simulink model "momentumBasedFlying"  (Simulink 9.0)
settings: Solver=FixedStepAuto  StartTime=0.0  StopTime="Config.simulationTime "  FixedStep=Config.Ts  RelTol=1e-3  EnableMultiTasking=on
InitFcn:
  | cd(fileparts(which(bdroot)));
  | initMomentumBasedFlying;
StopFcn:
  | visualizer_demo_idyntree(time.Data,state.Data,Config,desired_x_dx_ddx_dddx_CoM,jetsIntensitiesByWeight);
undefined symbols (not defined in the file or in its folder): Config, config
libraries: WBToolboxLibrary x67, simulink x2
(part 1 of 2)
settings Model: SuppressorTable=22 serialization::archive 11 0 6 0 0 0 11 0  Creator=DanielePucci  LastModifiedBy=gnava
settings DataIOCC: LimitDataPoints=on  SaveFormat=Dataset
settings DebuggingCC: UnderspecifiedInitializationDetection=Simplified  MergeDetectMultiDrivingBlocksExec=error  AllowSymbolicDim=off
settings HardwareCC: ProdBitPerPointer=64  ProdBitPerSizeT=64  ProdBitPerPtrDiffT=64  ProdLargestAtomicFloat=Float  ProdIntDivRoundTo=Zero  ProdEndianess=LittleEndian  ProdWordSize=64  ProdHWDeviceType=Intel->x86-64 (Windows64)

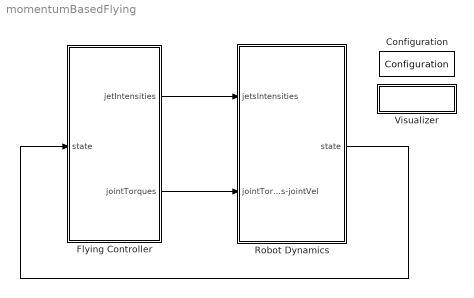
== system momentumBasedFlying ==
  Configuration : WBToolboxLibrary/Utilities/Configuration  ConfigSource=Workspace  ConfigObject='WBTConfigRobot'
      settings: SourceProductName=Whole Body Toolbox
  Flying Controller : Subsystem
  Robot Dynamics : Subsystem
  Visualizer : Subsystem
      mask Display: disp('Visualizer');
  wires:
  Flying Controller/1(jetIntensities) -> Robot Dynamics/1(jetsIntensities)
  Flying Controller/2(jointTorques) -> Robot Dynamics/2(jointTorques-jointVel)
  Robot Dynamics/1(state) -> Flying Controller/1(state)

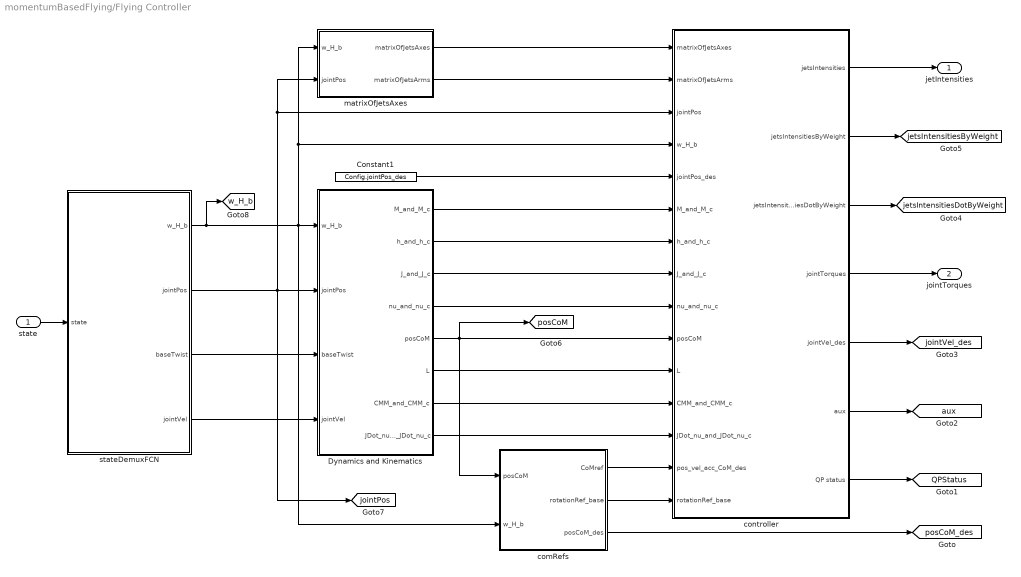
== system momentumBasedFlying/Flying Controller ==
  state : Inport
  Constant1 : Constant  Value=Config.jointPos_des
  Dynamics and Kinematics : Subsystem
  comRefs : Subsystem
  controller : Subsystem
  matrixOfJetsAxes : Subsystem
  stateDemuxFCN : MATLAB Function  TreatAsAtomicUnit=on
  jetIntensities : Outport
  jointTorques : Outport  Port=2
  tag scope: QPStatus=global, aux=global, jetsIntensitiesByWeight=global, jetsIntensitiesDotByWeight=global, jointPos=global, jointVel_des=global, posCoM=global, posCoM_des=global, w_H_b=global
  wires:
  state/1 -> stateDemuxFCN/1(state)
  controller/4(jointTorques) -> jointTorques/1
  controller/1(jetsIntensities) -> jetIntensities/1
  stateDemuxFCN/4(jointVel) -> Dynamics and Kinematics/4(jointVel)
  stateDemuxFCN/3(baseTwist) -> Dynamics and Kinematics/3(baseTwist)
  stateDemuxFCN/2(jointPos) -> [jointPos], matrixOfJetsAxes/2(jointPos), controller/3(jointPos), Dynamics and Kinematics/2(jointPos)
  stateDemuxFCN/1(w_H_b) -> comRefs/2(w_H_b), matrixOfJetsAxes/1(w_H_b), controller/4(w_H_b), Dynamics and Kinematics/1(w_H_b), [w_H_b]
  Dynamics and Kinematics/1(M_and_M_c) -> controller/6(M_and_M_c)
  Dynamics and Kinematics/2(h_and_h_c) -> controller/7(h_and_h_c)
  Dynamics and Kinematics/3(J_and_J_c) -> controller/8(J_and_J_c)
  Dynamics and Kinematics/4(nu_and_nu_c) -> controller/9(nu_and_nu_c)
  Dynamics and Kinematics/5(posCoM) -> [posCoM], comRefs/1(posCoM), controller/10(posCoM)
  Dynamics and Kinematics/6(L) -> controller/11(L)
  Dynamics and Kinematics/7(CMM_and_CMM_c) -> controller/12(CMM_and_CMM_c)
  Dynamics and Kinematics/8(JDot_nu_and_JDot_nu_c) -> controller/13(JDot_nu_and_JDot_nu_c)
  matrixOfJetsAxes/1(matrixOfJetsAxes) -> controller/1(matrixOfJetsAxes)
  matrixOfJetsAxes/2(matrixOfJetsArms) -> controller/2(matrixOfJetsArms)
  Constant1/1 -> controller/5(jointPos_des)
  comRefs/1(CoMref) -> controller/14(pos_vel_acc_CoM_des)
  comRefs/2(rotationRef_base) -> controller/15(rotationRef_base)
  comRefs/3(posCoM_des) -> [posCoM_des]
  controller/2(jetsIntensitiesByWeight) -> [jetsIntensitiesByWeight]
  controller/3(jetsIntensitiesDotByWeight) -> [jetsIntensitiesDotByWeight]
  controller/5(jointVel_des) -> [jointVel_des]
  controller/6(aux) -> [aux]
  controller/7(QP status) -> [QPStatus]

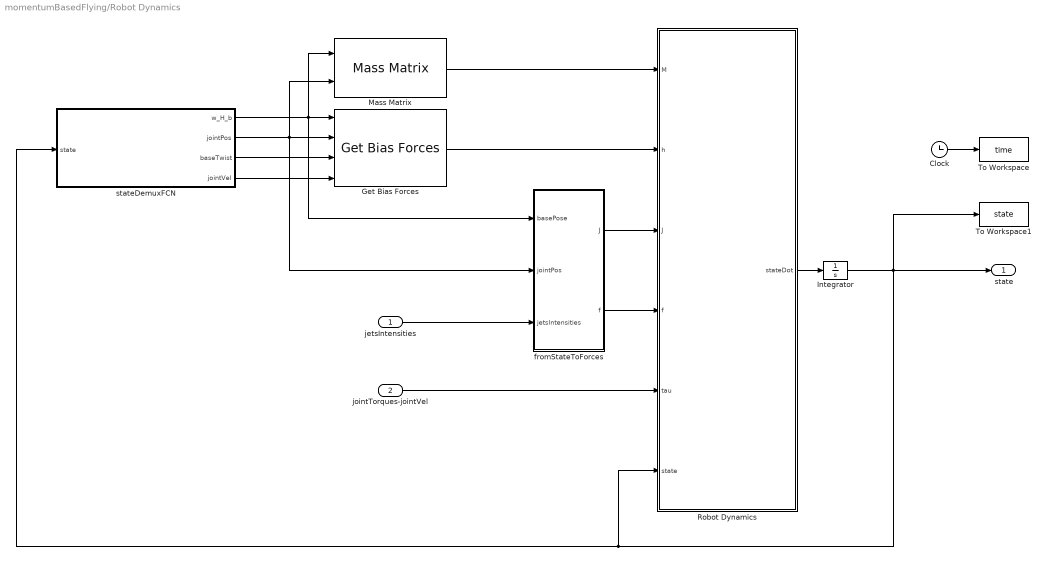
== system momentumBasedFlying/Robot Dynamics ==
  jetsIntensities : Inport
  jointTorques-jointVel : Inport  Port=2
  Clock : Clock
  Get Bias Forces : WBToolboxLibrary/wholeBodyModel/Dynamics/Get Bias Forces
      settings: SourceProductName=Whole Body Toolbox
  Integrator : Integrator  InitialCondition=Config.initState
  Mass Matrix : WBToolboxLibrary/wholeBodyModel/Dynamics/Mass Matrix
      settings: SourceProductName=Whole Body Toolbox
  Robot Dynamics : MATLAB Function  TreatAsAtomicUnit=on
  To Workspace : ToWorkspace  VariableName=time  SaveFormat=Timeseries  SampleTime=-1
  To Workspace1 : ToWorkspace  VariableName=state  SaveFormat=Timeseries  SampleTime=-1
  fromStateToForces : Subsystem
  stateDemuxFCN : MATLAB Function  TreatAsAtomicUnit=on
  state : Outport
  wires:
  Robot Dynamics/1(stateDot) -> Integrator/1
  jointTorques-jointVel/1 -> Robot Dynamics/5(tau)
  stateDemuxFCN/4(jointVel) -> Get Bias Forces/4
  stateDemuxFCN/2(jointPos) -> fromStateToForces/2(jointPos), Get Bias Forces/2, Mass Matrix/2
  stateDemuxFCN/1(w_H_b) -> fromStateToForces/1(basePose), Get Bias Forces/1, Mass Matrix/1
  stateDemuxFCN/3(baseTwist) -> Get Bias Forces/3
  Mass Matrix/1 -> Robot Dynamics/1(M)
  Get Bias Forces/1 -> Robot Dynamics/2(h)
  jetsIntensities/1 -> fromStateToForces/3(jetsIntensities)
  fromStateToForces/1(J) -> Robot Dynamics/3(J)
  fromStateToForces/2(f) -> Robot Dynamics/4(f)
  Integrator/1 -> To Workspace1/1, state/1, Robot Dynamics/6(state), stateDemuxFCN/1(state)
  Clock/1 -> To Workspace/1

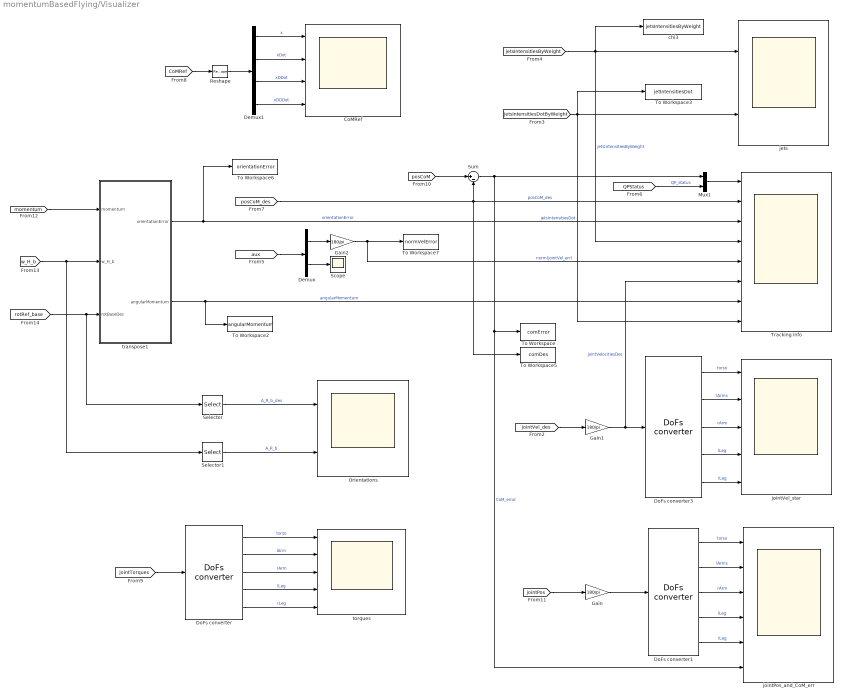
== system momentumBasedFlying/Visualizer ==
  CoMRef : Scope  NumInputPorts=4
  Demux : Demux  Outputs=2
  Demux1 : Demux  Outputs=[3;3;3;3]
  DoFs converter : WBToolboxLibrary/Utilities/DoFs converter  yarp2WBIOption=From YARP to WBI
      settings: SourceProductName=Whole Body Toolbox
  DoFs converter1 : WBToolboxLibrary/Utilities/DoFs converter  yarp2WBIOption=From YARP to WBI
      settings: SourceProductName=Whole Body Toolbox
  DoFs converter3 : WBToolboxLibrary/Utilities/DoFs converter  yarp2WBIOption=From YARP to WBI
      settings: SourceProductName=Whole Body Toolbox
  Gain : Gain  Gain=180/pi
  Gain1 : Gain  Gain=180/pi
  Gain2 : Gain  Gain=180/pi
  Mux1 : Mux  Inputs=2
  Orientations : Scope  NumInputPorts=2
  Reshape : Reshape
  Scope : Scope
  Selector : Selector  NumberOfDimensions=2  InputPortWidth=3  IndexOptions=Index vector (dialog),Index vector (dialog)  Indices=[1 2 3],[1 2 3]  OutputSizes=1,1
  Selector1 : Selector  NumberOfDimensions=2  InputPortWidth=3  IndexOptions=Index vector (dialog),Index vector (dialog)  Indices=[1 2 3],[1 2 3]  OutputSizes=1,1
  Sum : Sum  Inputs=|+-
  To Workspace : ToWorkspace  VariableName=comError  SaveFormat=Timeseries  SampleTime=-1
  To Workspace2 : ToWorkspace  VariableName=angularMomentum  SaveFormat=Timeseries  SampleTime=-1
  To Workspace3 : ToWorkspace  VariableName=jetIntensitiesDot  SaveFormat=Timeseries  SampleTime=-1
  To Workspace5 : ToWorkspace  VariableName=comDes  SaveFormat=Timeseries  SampleTime=-1
  To Workspace6 : ToWorkspace  VariableName=orientationError  SaveFormat=Timeseries  SampleTime=-1
  To Workspace7 : ToWorkspace  VariableName=normVelError  SaveFormat=Timeseries  SampleTime=-1
  Tracking info : Scope  NumInputPorts=8
  chi3 : ToWorkspace  VariableName=jetsIntensitiesByWeight  SaveFormat=Timeseries  SampleTime=-1
  jets : Scope  NumInputPorts=2
  jointPos_and_CoM_err : Scope  NumInputPorts=6
  jointVel_star : Scope  NumInputPorts=5
  torques : Scope  NumInputPorts=5
  transpose1 : MATLAB Function  TreatAsAtomicUnit=on
  wires:
  Demux/1 -> Gain2/1
  DoFs converter1/5 -> jointPos_and_CoM_err/5  "rLeg"
  DoFs converter/2 -> torques/2  "lArm"
  Mux1/1 -> Tracking info/1
  DoFs converter/1 -> torques/1  "torso"
  DoFs converter/5 -> torques/5  "rLeg"
  DoFs converter/3 -> torques/3  "rArm"
  DoFs converter1/3 -> jointPos_and_CoM_err/3  "rArm"
  Gain1/1 -> Tracking info/6, DoFs converter3/1  "jointVelocitiesDes"
  DoFs converter1/1 -> jointPos_and_CoM_err/1  "torso"
  [jointVel_des] -> Gain1/1
  DoFs converter3/3 -> jointVel_star/3  "rArm"
  Gain2/1 -> Tracking info/5, To Workspace7/1  "norm(jointVel_err)"
  Demux/2 -> Scope/1
  transpose1/1(orientationError) -> To Workspace6/1, Tracking info/3  "orientationError"
  Gain/1 -> DoFs converter1/1
  [aux] -> Demux/1
  DoFs converter3/1 -> jointVel_star/1  "torso"
  [jetsIntensitiesDotByWeight] -> Tracking info/8, jets/2, To Workspace3/1  "jetsIntensitiesDot"
  [jetsIntensitiesByWeight] -> Tracking info/4, chi3/1, jets/1  "jetsIntensitiesByWeight"
  DoFs converter3/2 -> jointVel_star/2  "lArms"
  DoFs converter/4 -> torques/4  "lLeg"
  [jointTorques] -> DoFs converter/1
  transpose1/2(angularMomentum) -> Tracking info/7, To Workspace2/1  "angularMomentum"
  DoFs converter3/4 -> jointVel_star/4  "lLeg"
  DoFs converter1/2 -> jointPos_and_CoM_err/2  "lArms"
  Sum/1 -> Mux1/1, jointPos_and_CoM_err/6, To Workspace/1  "CoM_error"
  DoFs converter1/4 -> jointPos_and_CoM_err/4  "lLeg"
  DoFs converter3/5 -> jointVel_star/5  "rLeg"
  [QPStatus] -> Mux1/2  "QP_status"
  Selector/1 -> Orientations/1  "A_R_b_des"
  [rotRef_base] -> Selector/1, transpose1/3(rotBaseDes)
  [w_H_b] -> Selector1/1, transpose1/2(w_H_b)
  Selector1/1 -> Orientations/2  "A_R_b"
  Demux1/4 -> CoMRef/4  "xDDDot"
  Demux1/2 -> CoMRef/2  "xDot"
  Demux1/3 -> CoMRef/3  "xDDot"
  Demux1/1 -> CoMRef/1  "x"
  [posCoM_des] -> Sum/2, To Workspace5/1, Tracking info/2  "posCoM_des"
  [CoMRef] -> Reshape/1
  Reshape/1 -> Demux1/1
  [posCoM] -> Sum/1
  [jointPos] -> Gain/1
  [momentum] -> transpose1/1(momentum)

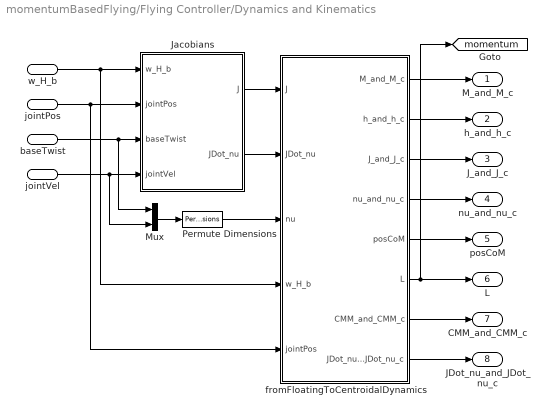
== system momentumBasedFlying/Flying Controller/Dynamics and Kinematics ==
  w_H_b : Inport
  jointPos : Inport  Port=2
  baseTwist : Inport  Port=3
  jointVel : Inport  Port=4
  Jacobians : Subsystem
  Mux : Mux  Inputs=2
  Permute Dimensions : PermuteDimensions
  fromFloatingToCentroidalDynamics : Subsystem
  M_and_M_c : Outport
  h_and_h_c : Outport  Port=2
  J_and_J_c : Outport  Port=3
  nu_and_nu_c : Outport  Port=4
  posCoM : Outport  Port=5
  L : Outport  Port=6
  CMM_and_CMM_c : Outport  Port=7
  JDot_nu_and_JDot_nu_c : Outport  Port=8
  tag scope: momentum=global
  wires:
  w_H_b/1 -> fromFloatingToCentroidalDynamics/4(w_H_b), Jacobians/1(w_H_b)
  jointPos/1 -> fromFloatingToCentroidalDynamics/5(jointPos), Jacobians/2(jointPos)
  jointVel/1 -> Mux/2, Jacobians/4(jointVel)
  baseTwist/1 -> Mux/1, Jacobians/3(baseTwist)
  Jacobians/1(J) -> fromFloatingToCentroidalDynamics/1(J)
  Mux/1 -> Permute Dimensions/1
  Jacobians/2(JDot_nu) -> fromFloatingToCentroidalDynamics/2(JDot_nu)
  Permute Dimensions/1 -> fromFloatingToCentroidalDynamics/3(nu)
  fromFloatingToCentroidalDynamics/2("h_and_h_c ") -> h_and_h_c/1
  fromFloatingToCentroidalDynamics/1(M_and_M_c) -> M_and_M_c/1
  fromFloatingToCentroidalDynamics/3(J_and_J_c) -> J_and_J_c/1
  fromFloatingToCentroidalDynamics/4(nu_and_nu_c) -> nu_and_nu_c/1
  fromFloatingToCentroidalDynamics/5(posCoM) -> posCoM/1
  fromFloatingToCentroidalDynamics/6(L) -> L/1, [momentum]
  fromFloatingToCentroidalDynamics/7(CMM_and_CMM_c) -> CMM_and_CMM_c/1
  fromFloatingToCentroidalDynamics/8(JDot_nu_and_JDot_nu_c) -> JDot_nu_and_JDot_nu_c/1

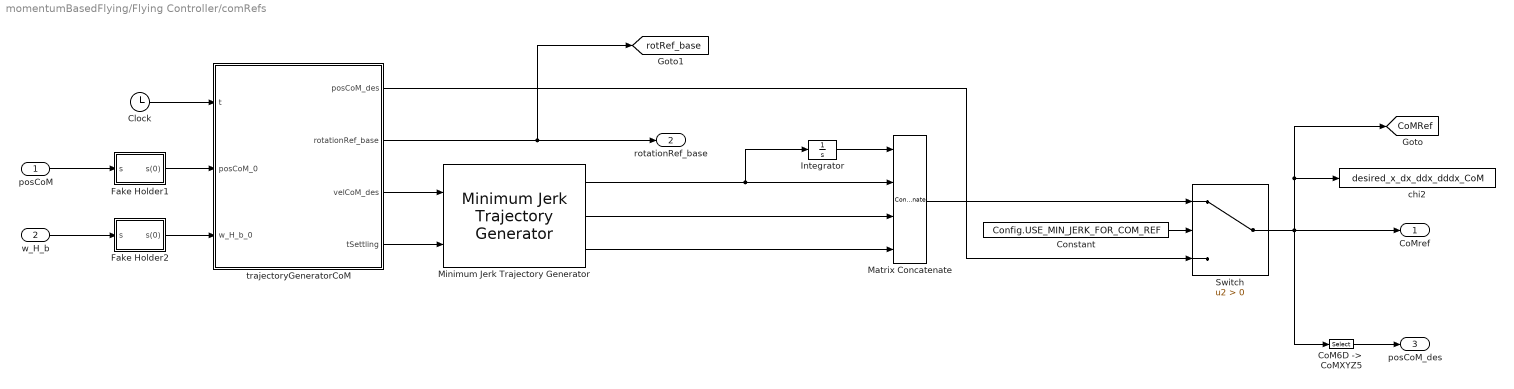
== system momentumBasedFlying/Flying Controller/comRefs ==
  posCoM : Inport
  w_H_b : Inport  Port=2
  Clock : Clock
  "CoM6D ->  CoMXYZ5" : Selector  NumberOfDimensions=2  InputPortWidth=7  IndexOptions=Index vector (dialog),Index vector (dialog)  Indices=[1 2 3],[1]  OutputSizes=1,1
  Constant : Constant  Value=Config.USE_MIN_JERK_FOR_COM_REF
  Fake Holder1 : Subsystem
  Fake Holder2 : Subsystem
  Integrator : Integrator  InitialCondition=Config.posCoM_des_0
  Matrix Concatenate : Concatenate  NumInputs=4  Mode=Multidimensional array  ConcatenateDimension=2
  Minimum Jerk Trajectory Generator : WBToolboxLibrary/Utilities/Minimum Jerk Trajectory Generator  externalSettlingTime=on  settlingTime=3  sampleTime=Config.Ts  resetOnSettlingTime=off  firstDerivatives=on  secondDerivatives=on  explicitInitialValue=off
      settings: SourceProductName=Whole Body Toolbox
  Switch : Switch  Criteria=u2 > Threshold
  chi2 : ToWorkspace  VariableName=desired_x_dx_ddx_dddx_CoM  SaveFormat=Timeseries  SampleTime=-1
  trajectoryGeneratorCoM : MATLAB Function  TreatAsAtomicUnit=on
  CoMref : Outport
  rotationRef_base : Outport  Port=2
  posCoM_des : Outport  Port=3
  tag scope: CoMRef=global, rotRef_base=global
  wires:
  Clock/1 -> trajectoryGeneratorCoM/1(t)
  trajectoryGeneratorCoM/1(posCoM_des) -> Switch/3
  posCoM/1 -> Fake Holder1/1(s)
  Fake Holder1/1(s(0)) -> trajectoryGeneratorCoM/2(posCoM_0)
  w_H_b/1 -> Fake Holder2/1(s)
  trajectoryGeneratorCoM/2(rotationRef_base) -> rotationRef_base/1, [rotRef_base]
  Fake Holder2/1(s(0)) -> trajectoryGeneratorCoM/3(w_H_b_0)
  trajectoryGeneratorCoM/3(velCoM_des) -> Minimum Jerk Trajectory Generator/1
  trajectoryGeneratorCoM/4(tSettling) -> Minimum Jerk Trajectory Generator/2
  Integrator/1 -> Matrix Concatenate/1
  Minimum Jerk Trajectory Generator/1 -> Integrator/1, Matrix Concatenate/2
  Minimum Jerk Trajectory Generator/2 -> Matrix Concatenate/3
  Minimum Jerk Trajectory Generator/3 -> Matrix Concatenate/4
  Matrix Concatenate/1 -> Switch/1
  Switch/1 -> [CoMRef], chi2/1, CoMref/1, "CoM6D ->  CoMXYZ5"/1
  Constant/1 -> Switch/2
  "CoM6D ->  CoMXYZ5"/1 -> posCoM_des/1

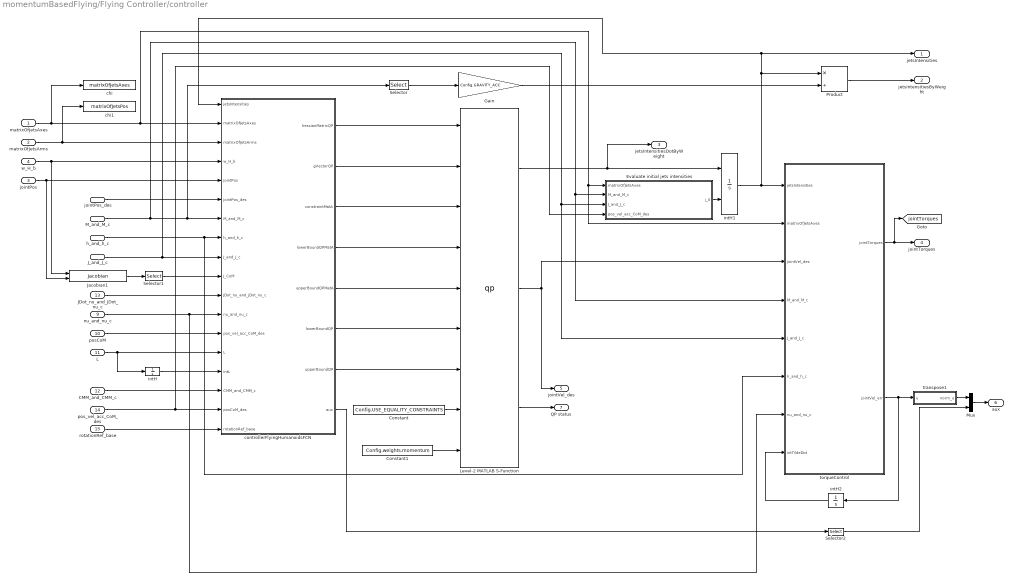
== system momentumBasedFlying/Flying Controller/controller ==
  matrixOfJetsAxes : Inport
  matrixOfJetsArms : Inport  Port=2
  jointPos : Inport  Port=3
  w_H_b : Inport  Port=4
  jointPos_des : Inport  Port=5
  M_and_M_c : Inport  Port=6
  h_and_h_c : Inport  Port=7
  J_and_J_c : Inport  Port=8
  nu_and_nu_c : Inport  Port=9
  posCoM : Inport  Port=10
  L : Inport  Port=11
  CMM_and_CMM_c : Inport  Port=12
  JDot_nu_and_JDot_nu_c : Inport  Port=13
  pos_vel_acc_CoM_des : Inport  Port=14
  rotationRef_base : Inport  Port=15
  Constant : Constant  Value=Config.USE_EQUALITY_CONSTRAINTS
  Constant1 : Constant  Value=Config.weights.momentum
  Evaluate initial jets intensities : MATLAB Function  TreatAsAtomicUnit=on
  Gain : Gain  Gain=Config.GRAVITY_ACC
  Jacobian1 : WBToolboxLibrary/wholeBodyModel/Jacobians/Jacobian  frameName=Frames.COM_FRAME
      settings: SourceProductName=Whole Body Toolbox
  Level-2 MATLAB S-Function : M-S-Function  FunctionName=qp  Parameters=Config.N_DOF  mask{ndof=Config.N_DOF}
      mask prompts: ndof "Robt degrees of freedom"
      mask Display: disp('QP')
  Mux : Mux  Inputs=2
  Product : Product  Inputs=*/
  Selector : Selector  NumberOfDimensions=2  InputPortWidth=3  IndexOptions=Index vector (dialog),Index vector (dialog)  Indices=1,1  OutputSizes=1,1
  Selector1 : Selector  NumberOfDimensions=2  InputPortWidth=3  IndexOptions=Index vector (dialog),Index vector (dialog)  Indices=[1 2 3],[1:Config.N_DOF+6]  OutputSizes=1,1
  Selector2 : Selector  InputPortWidth=2  IndexOptions=Index vector (dialog)  Indices=[2]  OutputSizes=1
  chi : ToWorkspace  VariableName=matrixOfJetsAxes  SaveFormat=Timeseries  SampleTime=-1
  chi1 : ToWorkspace  VariableName=matrixOfJetsPos  SaveFormat=Timeseries  SampleTime=-1
  controllerFlyingHumanoidsFCN : MATLAB Function  TreatAsAtomicUnit=on
  intH : Integrator  InitialCondition=zeros(6,1)
  intH1 : Integrator  InitialConditionSource=external  InitialCondition=config.jetsIntensities0
  intH2 : Integrator  InitialCondition=zeros(Config.N_DOF,1)
  torqueControl : MATLAB Function  TreatAsAtomicUnit=on
  transpose1 : MATLAB Function  TreatAsAtomicUnit=on
  jetsIntensities : Outport
  jetsIntensitiesByWeight : Outport  Port=2
  jetsIntensitiesDotByWeight : Outport  Port=3
  jointTorques : Outport  Port=4
  jointVel_des : Outport  Port=5
  aux : Outport  Port=6
  QP status : Outport  Port=7
  tag scope: jointTorques=global
  wires:
  Selector/1 -> Gain/1
  Product/1 -> jetsIntensitiesByWeight/1
  Gain/1 -> Product/2
  intH1/1 -> torqueControl/1(jetsIntensities), controllerFlyingHumanoidsFCN/1(jetsIntensities), jetsIntensities/1, Product/1
  controllerFlyingHumanoidsFCN/8(aux) -> Selector2/1
  Evaluate initial jets intensities/1(j_0) -> intH1/2
  torqueControl/1(jointTorques) -> [jointTorques], jointTorques/1
  Level-2 MATLAB S-Function/1 -> intH1/1, jetsIntensitiesDotByWeight/1
  intH2/1 -> torqueControl/8(intTildeDot)
  torqueControl/2(jointVel_err) -> intH2/1, transpose1/1(u)
  Level-2 MATLAB S-Function/2 -> jointVel_des/1, torqueControl/3(jointVel_des)
  Level-2 MATLAB S-Function/3 -> QP status/1
  Constant/1 -> Level-2 MATLAB S-Function/8
  Constant1/1 -> Level-2 MATLAB S-Function/9
  Jacobian1/1 -> Selector1/1
  Selector1/1 -> controllerFlyingHumanoidsFCN/10(J_CoM)
  Mux/1 -> aux/1
  Selector2/1 -> Mux/2
  transpose1/1(norm_u) -> Mux/1
  matrixOfJetsAxes/1 -> chi/1, controllerFlyingHumanoidsFCN/2(matrixOfJetsAxes), torqueControl/2(matrixOfJetsAxes), Evaluate initial jets intensities/1(matrixOfJetsAxes)
  matrixOfJetsArms/1 -> chi1/1, controllerFlyingHumanoidsFCN/3(matrixOfJetsArms)
  w_H_b/1 -> controllerFlyingHumanoidsFCN/4(w_H_b), Jacobian1/1
  jointPos/1 -> controllerFlyingHumanoidsFCN/5(jointPos), Jacobian1/2
  jointPos_des/1 -> controllerFlyingHumanoidsFCN/6(jointPos_des)
  M_and_M_c/1 -> controllerFlyingHumanoidsFCN/7(M_and_M_c), Selector/1, torqueControl/4(M_and_M_c), Evaluate initial jets intensities/2(M_and_M_c)
  h_and_h_c/1 -> torqueControl/6(h_and_h_c), controllerFlyingHumanoidsFCN/8(h_and_h_c)
  J_and_J_c/1 -> controllerFlyingHumanoidsFCN/9(J_and_J_c), torqueControl/5(J_and_J_c), Evaluate initial jets intensities/3(J_and_J_c)
  JDot_nu_and_JDot_nu_c/1 -> controllerFlyingHumanoidsFCN/11(JDot_nu_and_JDot_nu_c)
  nu_and_nu_c/1 -> controllerFlyingHumanoidsFCN/12(nu_and_nu_c), torqueControl/7(nu_and_nu_c)
  posCoM/1 -> controllerFlyingHumanoidsFCN/13(pos_vel_acc_CoM_des)
  intH/1 -> controllerFlyingHumanoidsFCN/15(intL)
  L/1 -> controllerFlyingHumanoidsFCN/14(L), intH/1
  CMM_and_CMM_c/1 -> controllerFlyingHumanoidsFCN/16(CMM_and_CMM_c)
  pos_vel_acc_CoM_des/1 -> controllerFlyingHumanoidsFCN/17(posCoM_des), Evaluate initial jets intensities/4(pos_vel_acc_CoM_des)
  rotationRef_base/1 -> controllerFlyingHumanoidsFCN/18(rotationRef_base)
  controllerFlyingHumanoidsFCN/7(upperBoundQP) -> Level-2 MATLAB S-Function/7
  controllerFlyingHumanoidsFCN/6(lowerBoundQP) -> Level-2 MATLAB S-Function/6
  controllerFlyingHumanoidsFCN/5(upperBoundQPMatA) -> Level-2 MATLAB S-Function/5
  controllerFlyingHumanoidsFCN/4(lowerBoundQPMatA) -> Level-2 MATLAB S-Function/4
  controllerFlyingHumanoidsFCN/3(constraintMatA) -> Level-2 MATLAB S-Function/3
  controllerFlyingHumanoidsFCN/2(gVectorQP) -> Level-2 MATLAB S-Function/2
  controllerFlyingHumanoidsFCN/1(hessianMatrixQP) -> Level-2 MATLAB S-Function/1

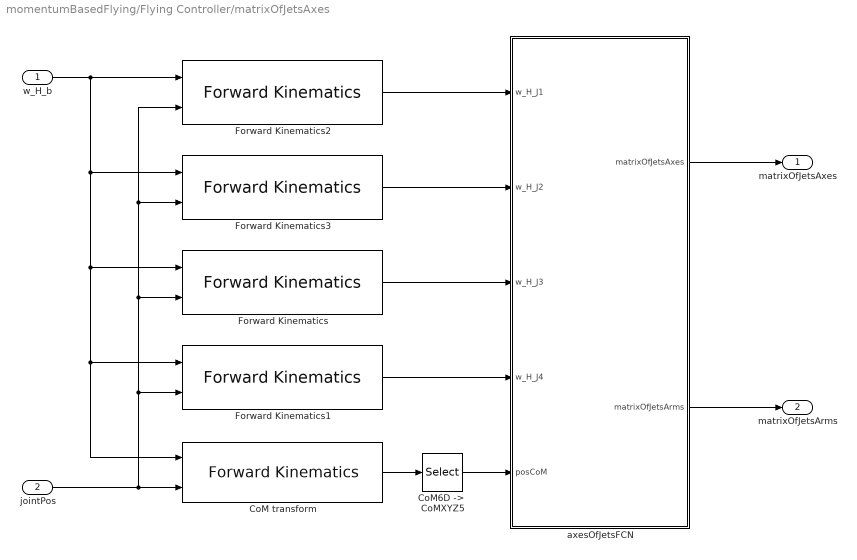
== system momentumBasedFlying/Flying Controller/matrixOfJetsAxes ==
  w_H_b : Inport
  jointPos : Inport  Port=2
  CoM transform : WBToolboxLibrary/wholeBodyModel/Kinematics/Forward Kinematics  frameName=Frames.COM_FRAME
      settings: SourceProductName=Whole Body Toolbox
  "CoM6D ->  CoMXYZ5" : Selector  NumberOfDimensions=2  InputPortWidth=7  IndexOptions=Index vector (dialog),Index vector (dialog)  Indices=[1 2 3],[4]  OutputSizes=1,1
  Forward Kinematics : WBToolboxLibrary/wholeBodyModel/Kinematics/Forward Kinematics  frameName=Frames.L_FOOT_FRAME
      settings: SourceProductName=Whole Body Toolbox
  Forward Kinematics1 : WBToolboxLibrary/wholeBodyModel/Kinematics/Forward Kinematics  frameName=Frames.R_FOOT_FRAME
      settings: SourceProductName=Whole Body Toolbox
  Forward Kinematics2 : WBToolboxLibrary/wholeBodyModel/Kinematics/Forward Kinematics  frameName=Frames.L_HAND_FRAME
      settings: SourceProductName=Whole Body Toolbox
  Forward Kinematics3 : WBToolboxLibrary/wholeBodyModel/Kinematics/Forward Kinematics  frameName=Frames.R_HAND_FRAME
      settings: SourceProductName=Whole Body Toolbox
  axesOfJetsFCN : MATLAB Function  TreatAsAtomicUnit=on
  matrixOfJetsAxes : Outport
  matrixOfJetsArms : Outport  Port=2
  wires:
  w_H_b/1 -> CoM transform/1, Forward Kinematics1/1, Forward Kinematics/1, Forward Kinematics3/1, Forward Kinematics2/1
  Forward Kinematics3/1 -> axesOfJetsFCN/2(w_H_J2)
  jointPos/1 -> Forward Kinematics2/2, Forward Kinematics3/2, Forward Kinematics/2, Forward Kinematics1/2, CoM transform/2
  Forward Kinematics2/1 -> axesOfJetsFCN/1(w_H_J1)
  Forward Kinematics/1 -> axesOfJetsFCN/3(w_H_J3)
  Forward Kinematics1/1 -> axesOfJetsFCN/4(w_H_J4)
  axesOfJetsFCN/1(matrixOfJetsAxes) -> matrixOfJetsAxes/1
  axesOfJetsFCN/2(matrixOfJetsArms) -> matrixOfJetsArms/1
  CoM transform/1 -> "CoM6D ->  CoMXYZ5"/1
  "CoM6D ->  CoMXYZ5"/1 -> axesOfJetsFCN/5(posCoM)

== system momentumBasedFlying/Robot Dynamics/fromStateToForces ==
  basePose : Inport
  jointPos : Inport  Port=2
  jetsIntensities : Inport  Port=3
  End Effectors Jacobians : Subsystem
  Terminator : Terminator
  fromJetsIntensitiesToForces : MATLAB Function  TreatAsAtomicUnit=on
  matrixOfJetsAxes : Subsystem
  J : Outport
  f : Outport  Port=2
  wires:
  jointPos/1 -> matrixOfJetsAxes/2(jointPos), End Effectors Jacobians/2(jointPos)
  basePose/1 -> End Effectors Jacobians/1(w_H_b), matrixOfJetsAxes/1(w_H_b)
  End Effectors Jacobians/1(J_EE) -> J/1
  fromJetsIntensitiesToForces/1(f) -> f/1
  jetsIntensities/1 -> fromJetsIntensitiesToForces/2(jetsIntensities)
  matrixOfJetsAxes/1(matrixOfJetsAxes) -> fromJetsIntensitiesToForces/1(matrixOfJetsAxes)
  matrixOfJetsAxes/2(matrixOfJetsArms) -> Terminator/1

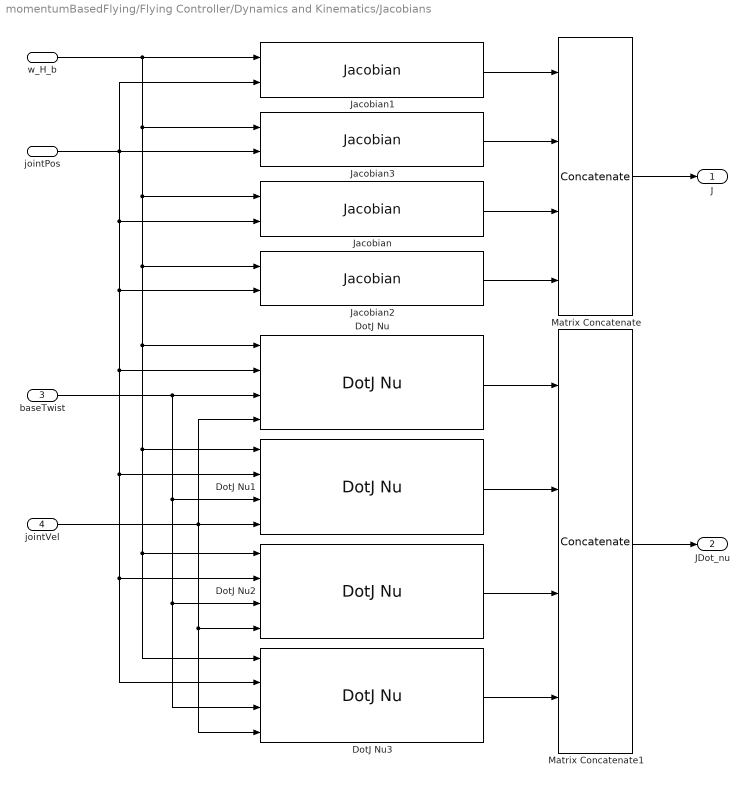
== system momentumBasedFlying/Flying Controller/Dynamics and Kinematics/Jacobians ==
  w_H_b : Inport
  jointPos : Inport  Port=2
  baseTwist : Inport  Port=3
  jointVel : Inport  Port=4
  DotJ Nu : WBToolboxLibrary/wholeBodyModel/Jacobians/DotJ Nu  frameName=Frames.L_HAND_FRAME
      settings: SourceProductName=Whole Body Toolbox
  DotJ Nu1 : WBToolboxLibrary/wholeBodyModel/Jacobians/DotJ Nu  frameName=Frames.R_HAND_FRAME
      settings: SourceProductName=Whole Body Toolbox
  DotJ Nu2 : WBToolboxLibrary/wholeBodyModel/Jacobians/DotJ Nu  frameName=Frames.L_FOOT_FRAME
      settings: SourceProductName=Whole Body Toolbox
  DotJ Nu3 : WBToolboxLibrary/wholeBodyModel/Jacobians/DotJ Nu  frameName=Frames.R_FOOT_FRAME
      settings: SourceProductName=Whole Body Toolbox
  Jacobian : WBToolboxLibrary/wholeBodyModel/Jacobians/Jacobian  frameName=Frames.L_FOOT_FRAME
      settings: SourceProductName=Whole Body Toolbox
  Jacobian1 : WBToolboxLibrary/wholeBodyModel/Jacobians/Jacobian  frameName=Frames.L_HAND_FRAME
      settings: SourceProductName=Whole Body Toolbox
  Jacobian2 : WBToolboxLibrary/wholeBodyModel/Jacobians/Jacobian  frameName=Frames.R_FOOT_FRAME
      settings: SourceProductName=Whole Body Toolbox
  Jacobian3 : WBToolboxLibrary/wholeBodyModel/Jacobians/Jacobian  frameName=Frames.R_HAND_FRAME
      settings: SourceProductName=Whole Body Toolbox
  Matrix Concatenate : Concatenate  NumInputs=4  Mode=Multidimensional array
  Matrix Concatenate1 : Concatenate  NumInputs=4  Mode=Multidimensional array
  J : Outport
  JDot_nu : Outport  Port=2
  wires:
  Matrix Concatenate/1 -> J/1
  w_H_b/1 -> Jacobian/1, Jacobian2/1, DotJ Nu/1, DotJ Nu3/1, DotJ Nu2/1, DotJ Nu1/1, Jacobian3/1, Jacobian1/1
  Jacobian1/1 -> Matrix Concatenate/1
  Jacobian3/1 -> Matrix Concatenate/2
  Jacobian/1 -> Matrix Concatenate/3
  Jacobian2/1 -> Matrix Concatenate/4
  jointPos/1 -> Jacobian2/2, DotJ Nu/2, DotJ Nu3/2, DotJ Nu2/2, DotJ Nu1/2, Jacobian/2, Jacobian3/2, Jacobian1/2
  baseTwist/1 -> DotJ Nu/3, DotJ Nu3/3, DotJ Nu2/3, DotJ Nu1/3
  jointVel/1 -> DotJ Nu3/4, DotJ Nu2/4, DotJ Nu/4, DotJ Nu1/4
  DotJ Nu/1 -> Matrix Concatenate1/1
  DotJ Nu1/1 -> Matrix Concatenate1/2
  DotJ Nu2/1 -> Matrix Concatenate1/3
  DotJ Nu3/1 -> Matrix Concatenate1/4
  Matrix Concatenate1/1 -> JDot_nu/1

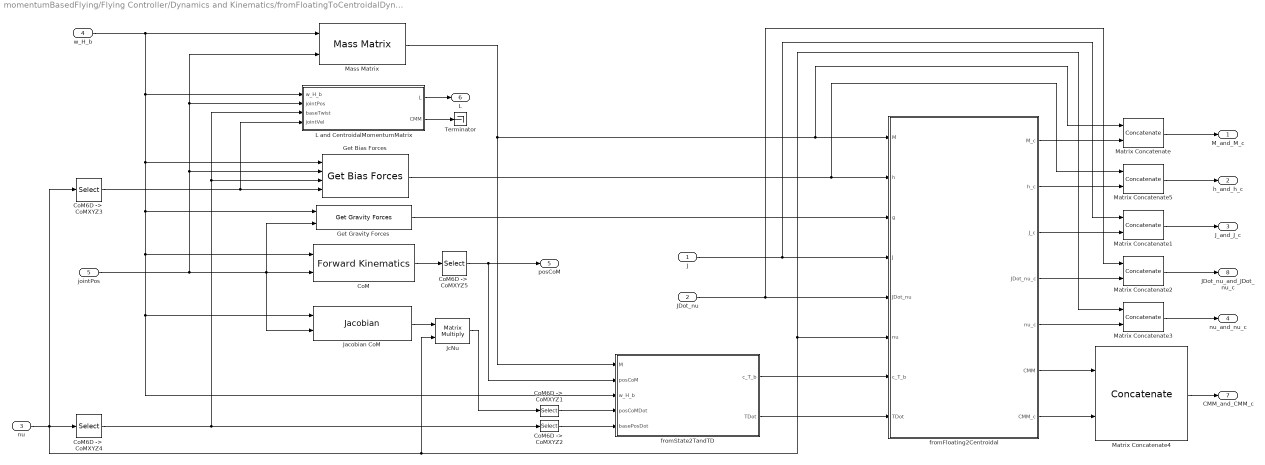
== system momentumBasedFlying/Flying Controller/Dynamics and Kinematics/fromFloatingToCentroidalDynamics ==
  J : Inport
  JDot_nu : Inport  Port=2
  nu : Inport  Port=3
  w_H_b : Inport  Port=4
  jointPos : Inport  Port=5
  CoM : WBToolboxLibrary/wholeBodyModel/Kinematics/Forward Kinematics  frameName=Frames.COM_FRAME
      settings: SourceProductName=Whole Body Toolbox
  "CoM6D ->  CoMXYZ1" : Selector  InputPortWidth=6  IndexOptions=Index vector (dialog)  Indices=[1 2 3]  OutputSizes=1
  "CoM6D ->  CoMXYZ2" : Selector  InputPortWidth=6  IndexOptions=Index vector (dialog)  Indices=[1 2 3]  OutputSizes=1
  "CoM6D ->  CoMXYZ3" : Selector  InputPortWidth=6+Config.N_DOF  IndexOptions=Index vector (dialog)  Indices=[7:6+Config.N_DOF]  OutputSizes=1
  "CoM6D ->  CoMXYZ4" : Selector  InputPortWidth=6+Config.N_DOF  IndexOptions=Index vector (dialog)  Indices=[1 2 3 4 5 6]  OutputSizes=1
  "CoM6D ->  CoMXYZ5" : Selector  NumberOfDimensions=2  InputPortWidth=7  IndexOptions=Index vector (dialog),Index vector (dialog)  Indices=[1 2 3],[4]  OutputSizes=1,1
  Get Bias Forces : WBToolboxLibrary/wholeBodyModel/Dynamics/Get Bias Forces
      settings: SourceProductName=Whole Body Toolbox
  Get Gravity Forces : WBToolboxLibrary/wholeBodyModel/Dynamics/Get Gravity Forces
      settings: SourceProductName=Whole Body Toolbox
  Jacobian CoM : WBToolboxLibrary/wholeBodyModel/Jacobians/Jacobian  frameName=Frames.COM_FRAME
      settings: SourceProductName=Whole Body Toolbox
  JcNu : Product  Multiplication=Matrix(*)
  L and CentroidalMomentumMatrix : Subsystem
  Mass Matrix : WBToolboxLibrary/wholeBodyModel/Dynamics/Mass Matrix
      settings: SourceProductName=Whole Body Toolbox
  Matrix Concatenate{,2..3,5} (4 alike) : Concatenate  Mode=Multidimensional array  ConcatenateDimension=2
  Matrix Concatenate1 : Concatenate  Mode=Multidimensional array
  Matrix Concatenate4 : Concatenate  Mode=Multidimensional array
  Terminator : Terminator
  fromFloating2Centroidal : MATLAB Function  TreatAsAtomicUnit=on
  fromState2TandTD : MATLAB Function  TreatAsAtomicUnit=on
  M_and_M_c : Outport
  "h_and_h_c " : Outport  Port=2
  J_and_J_c : Outport  Port=3
  nu_and_nu_c : Outport  Port=4
  posCoM : Outport  Port=5
  L : Outport  Port=6
  CMM_and_CMM_c : Outport  Port=7
  JDot_nu_and_JDot_nu_c : Outport  Port=8
  wires:
  w_H_b/1 -> CoM/1, fromState2TandTD/3(w_H_b), Jacobian CoM/1, Get Gravity Forces/1, Get Bias Forces/1, L and CentroidalMomentumMatrix/1(w_H_b), Mass Matrix/1
  jointPos/1 -> Mass Matrix/2, L and CentroidalMomentumMatrix/2(jointPos), Get Bias Forces/2, Jacobian CoM/2, CoM/2, Get Gravity Forces/2
  "CoM6D ->  CoMXYZ4"/1 -> L and CentroidalMomentumMatrix/3(baseTwist), Get Bias Forces/3, "CoM6D ->  CoMXYZ2"/1
  "CoM6D ->  CoMXYZ3"/1 -> L and CentroidalMomentumMatrix/4(jointVel), Get Bias Forces/4
  Mass Matrix/1 -> fromState2TandTD/1(M), fromFloating2Centroidal/1(M), Matrix Concatenate/1
  Get Bias Forces/1 -> fromFloating2Centroidal/2(h), Matrix Concatenate5/1
  Get Gravity Forces/1 -> fromFloating2Centroidal/3(g)
  J/1 -> fromFloating2Centroidal/4(J), Matrix Concatenate1/1
  JDot_nu/1 -> Matrix Concatenate2/1, fromFloating2Centroidal/5(JDot_nu)
  CoM/1 -> "CoM6D ->  CoMXYZ5"/1
  "CoM6D ->  CoMXYZ5"/1 -> posCoM/1, fromState2TandTD/2(posCoM)
  Jacobian CoM/1 -> JcNu/1
  JcNu/1 -> "CoM6D ->  CoMXYZ1"/1
  "CoM6D ->  CoMXYZ1"/1 -> fromState2TandTD/4(posCoMDot)
  fromState2TandTD/1(c_T_b) -> fromFloating2Centroidal/7(c_T_b)
  fromState2TandTD/2(TDot) -> fromFloating2Centroidal/8(TDot)
  "CoM6D ->  CoMXYZ2"/1 -> fromState2TandTD/5(basePosDot)
  nu/1 -> "CoM6D ->  CoMXYZ3"/1, fromFloating2Centroidal/6(nu), Matrix Concatenate3/1, JcNu/2, "CoM6D ->  CoMXYZ4"/1
  L and CentroidalMomentumMatrix/1(L) -> L/1
  Matrix Concatenate/1 -> M_and_M_c/1
  fromFloating2Centroidal/1(M_c) -> Matrix Concatenate/2
  fromFloating2Centroidal/2(h_c) -> Matrix Concatenate5/2
  Matrix Concatenate5/1 -> "h_and_h_c "/1
  Matrix Concatenate1/1 -> J_and_J_c/1
  fromFloating2Centroidal/3(J_c) -> Matrix Concatenate1/2
  Matrix Concatenate2/1 -> JDot_nu_and_JDot_nu_c/1
  fromFloating2Centroidal/4(JDot_nu_c) -> Matrix Concatenate2/2
  Matrix Concatenate3/1 -> nu_and_nu_c/1
  fromFloating2Centroidal/5(nu_c) -> Matrix Concatenate3/2
  Matrix Concatenate4/1 -> CMM_and_CMM_c/1
  fromFloating2Centroidal/7(CMM_c) -> Matrix Concatenate4/2
  fromFloating2Centroidal/6(CMM) -> Matrix Concatenate4/1
  L and CentroidalMomentumMatrix/2(CMM) -> Terminator/1

== system momentumBasedFlying/Flying Controller/comRefs/Fake Holder1 ==
  s : Inport
  Clock1 : Clock
  Compare To Constant : simulink/Logic and Bit Operations/Compare To Constant  relop===  const=0  OutDataTypeStr=boolean
  MATLAB Function : MATLAB Function  TreatAsAtomicUnit=on
  s(0) : Outport
  wires:
  Compare To Constant/1 -> MATLAB Function/2(unused)
  MATLAB Function/1(s0) -> s(0)/1
  Clock1/1 -> Compare To Constant/1
  s/1 -> MATLAB Function/1(s)

== system momentumBasedFlying/Flying Controller/comRefs/Fake Holder2 ==
  s : Inport
  Clock1 : Clock
  Compare To Constant : simulink/Logic and Bit Operations/Compare To Constant  relop===  const=0  OutDataTypeStr=boolean
  MATLAB Function : MATLAB Function  TreatAsAtomicUnit=on
  s(0) : Outport
  wires:
  Compare To Constant/1 -> MATLAB Function/2(unused)
  MATLAB Function/1(s0) -> s(0)/1
  Clock1/1 -> Compare To Constant/1
  s/1 -> MATLAB Function/1(s)

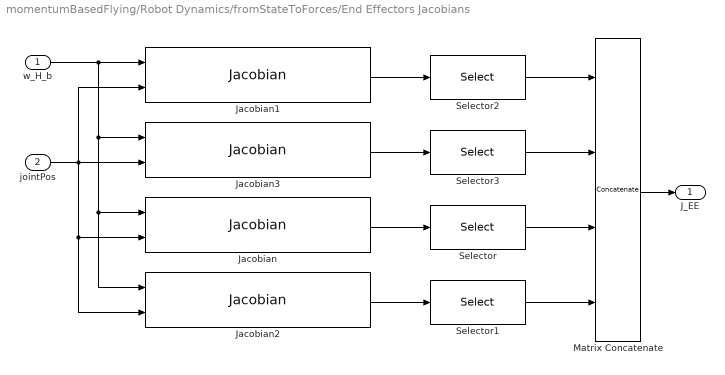
== system momentumBasedFlying/Robot Dynamics/fromStateToForces/End Effectors Jacobians ==
  w_H_b : Inport
  jointPos : Inport  Port=2
  Jacobian : WBToolboxLibrary/wholeBodyModel/Jacobians/Jacobian  frameName=Frames.L_FOOT_FRAME
      settings: SourceProductName=Whole Body Toolbox
  Jacobian1 : WBToolboxLibrary/wholeBodyModel/Jacobians/Jacobian  frameName=Frames.L_HAND_FRAME
      settings: SourceProductName=Whole Body Toolbox
  Jacobian2 : WBToolboxLibrary/wholeBodyModel/Jacobians/Jacobian  frameName=Frames.R_FOOT_FRAME
      settings: SourceProductName=Whole Body Toolbox
  Jacobian3 : WBToolboxLibrary/wholeBodyModel/Jacobians/Jacobian  frameName=Frames.R_HAND_FRAME
      settings: SourceProductName=Whole Body Toolbox
  Matrix Concatenate : Concatenate  NumInputs=4  Mode=Multidimensional array
  Selector{,1..3} (4 alike) : Selector  NumberOfDimensions=2  InputPortWidth=3  IndexOptions=Index vector (dialog),Index vector (dialog)  Indices=[1 2 3],[1:Config.N_DOF+6]  OutputSizes=1,1
  J_EE : Outport
  wires:
  Jacobian/1 -> Selector/1
  Jacobian2/1 -> Selector1/1
  w_H_b/1 -> Jacobian2/1, Jacobian/1, Jacobian3/1, Jacobian1/1
  jointPos/1 -> Jacobian2/2, Jacobian/2, Jacobian1/2, Jacobian3/2
  Jacobian1/1 -> Selector2/1
  Jacobian3/1 -> Selector3/1
  Selector1/1 -> Matrix Concatenate/4
  Matrix Concatenate/1 -> J_EE/1
  Selector3/1 -> Matrix Concatenate/2
  Selector2/1 -> Matrix Concatenate/1
  Selector/1 -> Matrix Concatenate/3

== system momentumBasedFlying/Robot Dynamics/fromStateToForces/matrixOfJetsAxes ==
  w_H_b : Inport
  jointPos : Inport  Port=2
  CoM transform : WBToolboxLibrary/wholeBodyModel/Kinematics/Forward Kinematics  frameName=Frames.COM_FRAME
      settings: SourceProductName=Whole Body Toolbox
  "CoM6D ->  CoMXYZ5" : Selector  NumberOfDimensions=2  InputPortWidth=7  IndexOptions=Index vector (dialog),Index vector (dialog)  Indices=[1 2 3],[4]  OutputSizes=1,1
  Forward Kinematics : WBToolboxLibrary/wholeBodyModel/Kinematics/Forward Kinematics  frameName=Frames.L_FOOT_FRAME
      settings: SourceProductName=Whole Body Toolbox
  Forward Kinematics1 : WBToolboxLibrary/wholeBodyModel/Kinematics/Forward Kinematics  frameName=Frames.R_FOOT_FRAME
      settings: SourceProductName=Whole Body Toolbox
  Forward Kinematics2 : WBToolboxLibrary/wholeBodyModel/Kinematics/Forward Kinematics  frameName=Frames.L_HAND_FRAME
      settings: SourceProductName=Whole Body Toolbox
  Forward Kinematics3 : WBToolboxLibrary/wholeBodyModel/Kinematics/Forward Kinematics  frameName=Frames.R_HAND_FRAME
      settings: SourceProductName=Whole Body Toolbox
  axesOfJetsFCN : MATLAB Function  TreatAsAtomicUnit=on
  matrixOfJetsAxes : Outport
  matrixOfJetsArms : Outport  Port=2
  wires:
  w_H_b/1 -> CoM transform/1, Forward Kinematics1/1, Forward Kinematics/1, Forward Kinematics3/1, Forward Kinematics2/1
  Forward Kinematics3/1 -> axesOfJetsFCN/2(w_H_J2)
  jointPos/1 -> Forward Kinematics2/2, Forward Kinematics3/2, Forward Kinematics/2, Forward Kinematics1/2, CoM transform/2
  Forward Kinematics2/1 -> axesOfJetsFCN/1(w_H_J1)
  Forward Kinematics/1 -> axesOfJetsFCN/3(w_H_J3)
  Forward Kinematics1/1 -> axesOfJetsFCN/4(w_H_J4)
  axesOfJetsFCN/1(matrixOfJetsAxes) -> matrixOfJetsAxes/1
  axesOfJetsFCN/2(matrixOfJetsArms) -> matrixOfJetsArms/1
  CoM transform/1 -> "CoM6D ->  CoMXYZ5"/1
  "CoM6D ->  CoMXYZ5"/1 -> axesOfJetsFCN/5(posCoM)

== system momentumBasedFlying/Flying Controller/Dynamics and Kinematics/fromFloatingToCentroidalDynamics/L and CentroidalMomentumMatrix ==
  w_H_b : Inport
  jointPos : Inport  Port=2
  baseTwist : Inport  Port=3
  jointVel : Inport  Port=4
  Centroidal Momentum : WBToolboxLibrary/wholeBodyModel/Dynamics/Centroidal Momentum
      settings: SourceProductName=Whole Body Toolbox
  "Centroidal Momentum Matrix " : Subsystem
  L : Outport
  CMM : Outport  Port=2
  wires:
  baseTwist/1 -> Centroidal Momentum/3
  Centroidal Momentum/1 -> L/1
  w_H_b/1 -> "Centroidal Momentum Matrix "/1(w_H_b), Centroidal Momentum/1
  jointPos/1 -> "Centroidal Momentum Matrix "/2(jointPos), Centroidal Momentum/2
  jointVel/1 -> Centroidal Momentum/4
  "Centroidal Momentum Matrix "/1(CMM) -> CMM/1

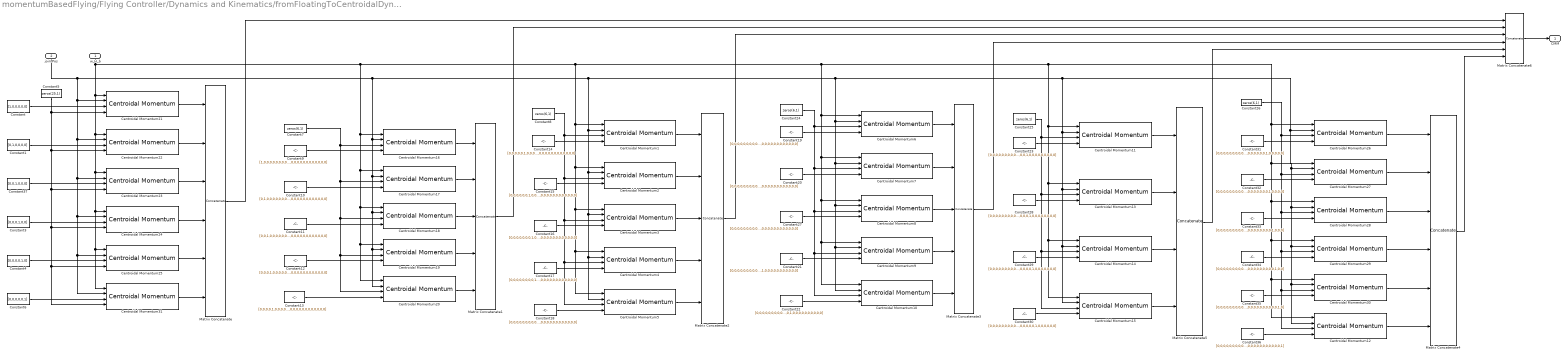
== system momentumBasedFlying/Flying Controller/Dynamics and Kinematics/fromFloatingToCentroidalDynamics/L and CentroidalMomentumMatrix/Centroidal Momentum Matrix  ==
  w_H_b : Inport
  jointPos : Inport  Port=2
  Centroidal Momentum{1..31} (31 alike) : WBToolboxLibrary/wholeBodyModel/Dynamics/Centroidal Momentum
      settings: SourceProductName=Whole Body Toolbox
  Constant : Constant  Value=[1,0,0,0,0,0]
  Constant1 : Constant  Value=[0,1,0,0,0,0]
  Constant10 : Constant  Value=[0,1,0,0,0,0,0,0,0,0,0,0,0,0,0,0,0,0,0,0,0,0,0,0,0]
  Constant11 : Constant  Value=[0,0,1,0,0,0,0,0,0,0,0,0,0,0,0,0,0,0,0,0,0,0,0,0,0]
  Constant12 : Constant  Value=[0,0,0,1,0,0,0,0,0,0,0,0,0,0,0,0,0,0,0,0,0,0,0,0,0]
  Constant13 : Constant  Value=[0,0,0,0,1,0,0,0,0,0,0,0,0,0,0,0,0,0,0,0,0,0,0,0,0]
  Constant14 : Constant  Value=[0,0,0,0,0,1,0,0,0,0,0,0,0,0,0,0,0,0,0,0,0,0,0,0,0]
  Constant15 : Constant  Value=[0,0,0,0,0,0,1,0,0,0,0,0,0,0,0,0,0,0,0,0,0,0,0,0,0]
  Constant16 : Constant  Value=[0,0,0,0,0,0,0,1,0,0,0,0,0,0,0,0,0,0,0,0,0,0,0,0,0]
  Constant17 : Constant  Value=[0,0,0,0,0,0,0,0,1,0,0,0,0,0,0,0,0,0,0,0,0,0,0,0,0]
  Constant18 : Constant  Value=[0,0,0,0,0,0,0,0,0,1,0,0,0,0,0,0,0,0,0,0,0,0,0,0,0]
  Constant19 : Constant  Value=[0,0,0,0,0,0,0,0,0,0,1,0,0,0,0,0,0,0,0,0,0,0,0,0,0]
  Constant20 : Constant  Value=[0,0,0,0,0,0,0,0,0,0,0,1,0,0,0,0,0,0,0,0,0,0,0,0,0]
  Constant21 : Constant  Value=[0,0,0,0,0,0,0,0,0,0,0,0,0,1,0,0,0,0,0,0,0,0,0,0,0]
  Constant22 : Constant  Value=[0,0,0,0,0,0,0,0,0,0,0,0,0,0,1,0,0,0,0,0,0,0,0,0,0]
  Constant23 : Constant  Value=[0,0,0,0,0,0,0,0,0,0,0,0,0,0,0,1,0,0,0,0,0,0,0,0,0]
  Constant{7..8,24..26} (5 alike) : Constant  Value=zeros(6,1)
  Constant27 : Constant  Value=[0,0,0,0,0,0,0,0,0,0,0,0,1,0,0,0,0,0,0,0,0,0,0,0,0]
  Constant28 : Constant  Value=[0,0,0,0,0,0,0,0,0,0,0,0,0,0,0,0,1,0,0,0,0,0,0,0,0]
  Constant29 : Constant  Value=[0,0,0,0,0,0,0,0,0,0,0,0,0,0,0,0,0,1,0,0,0,0,0,0,0]
  Constant3 : Constant  Value=[0,0,0,1,0,0]
  Constant30 : Constant  Value=[0,0,0,0,0,0,0,0,0,0,0,0,0,0,0,0,0,0,1,0,0,0,0,0,0]
  Constant31 : Constant  Value=[0,0,0,0,0,0,0,0,0,0,0,0,0,0,0,0,0,0,0,1,0,0,0,0,0]
  Constant32 : Constant  Value=[0,0,0,0,0,0,0,0,0,0,0,0,0,0,0,0,0,0,0,0,1,0,0,0,0]
  Constant33 : Constant  Value=[0,0,0,0,0,0,0,0,0,0,0,0,0,0,0,0,0,0,0,0,0,1,0,0,0]
  Constant34 : Constant  Value=[0,0,0,0,0,0,0,0,0,0,0,0,0,0,0,0,0,0,0,0,0,0,1,0,0]
  Constant35 : Constant  Value=[0,0,0,0,0,0,0,0,0,0,0,0,0,0,0,0,0,0,0,0,0,0,0,1,0]
  Constant36 : Constant  Value=[0,0,0,0,0,0,0,0,0,0,0,0,0,0,0,0,0,0,0,0,0,0,0,0,1]
  Constant37 : Constant  Value=[0,0,1,0,0,0]
  Constant4 : Constant  Value=[0,0,0,0,1,0]
  Constant5 : Constant  Value=zeros(25,1)
  Constant6 : Constant  Value=[0,0,0,0,0,1]
  Constant9 : Constant  Value=[1,0,0,0,0,0,0,0,0,0,0,0,0,0,0,0,0,0,0,0,0,0,0,0,0]
  Matrix Concatenate : Concatenate  NumInputs=6  Mode=Multidimensional array  ConcatenateDimension=2
  Matrix Concatenate1 : Concatenate  NumInputs=5  Mode=Multidimensional array  ConcatenateDimension=2
  Matrix Concatenate2 : Concatenate  NumInputs=5  Mode=Multidimensional array  ConcatenateDimension=2
  Matrix Concatenate3 : Concatenate  NumInputs=5  Mode=Multidimensional array  ConcatenateDimension=2
  Matrix Concatenate4 : Concatenate  NumInputs=6  Mode=Multidimensional array  ConcatenateDimension=2
  Matrix Concatenate5 : Concatenate  NumInputs=4  Mode=Multidimensional array  ConcatenateDimension=2
  Matrix Concatenate6 : Concatenate  NumInputs=6  Mode=Multidimensional array  ConcatenateDimension=2
  CMM : Outport
  wires:
  Centroidal Momentum19/1 -> Matrix Concatenate1/4
  Centroidal Momentum4/1 -> Matrix Concatenate2/4
  Centroidal Momentum25/1 -> Matrix Concatenate/5
  Matrix Concatenate/1 -> Matrix Concatenate6/1
  Centroidal Momentum12/1 -> Matrix Concatenate4/6
  Centroidal Momentum5/1 -> Matrix Concatenate2/5
  Centroidal Momentum23/1 -> Matrix Concatenate/3
  w_H_b/1 -> Centroidal Momentum12/1, Centroidal Momentum30/1, Centroidal Momentum29/1, Centroidal Momentum28/1, Centroidal Momentum27/1, Centroidal Momentum26/1, Centroidal Momentum15/1, Centroidal Momentum14/1, Centroidal Momentum13/1, Centroidal Momentum11/1, Centroidal Momentum10/1, Centroidal Momentum9/1, Centroidal Momentum8/1, Centroidal Momentum7/1, Centroidal Momentum6/1, Centroidal Momentum1/1, Centroidal Momentum5/1, Centroidal Momentum4/1, Centroidal Momentum3/1, Centroidal Momentum2/1, Centroidal Momentum16/1, Centroidal Momentum20/1, Centroidal Momentum19/1, Centroidal Momentum18/1, Centroidal Momentum17/1, Centroidal Momentum31/1, Centroidal Momentum25/1, Centroidal Momentum24/1, Centroidal Momentum23/1, Centroidal Momentum22/1, Centroidal Momentum21/1
  Matrix Concatenate5/1 -> Matrix Concatenate6/5
  Centroidal Momentum3/1 -> Matrix Concatenate2/3
  Centroidal Momentum29/1 -> Matrix Concatenate4/4
  Matrix Concatenate4/1 -> Matrix Concatenate6/6
  Centroidal Momentum24/1 -> Matrix Concatenate/4
  Centroidal Momentum2/1 -> Matrix Concatenate2/2
  Centroidal Momentum1/1 -> Matrix Concatenate2/1
  Matrix Concatenate1/1 -> Matrix Concatenate6/2
  Centroidal Momentum28/1 -> Matrix Concatenate4/3
  Centroidal Momentum15/1 -> Matrix Concatenate5/4
  Centroidal Momentum7/1 -> Matrix Concatenate3/2
  Centroidal Momentum14/1 -> Matrix Concatenate5/3
  Centroidal Momentum26/1 -> Matrix Concatenate4/1
  Centroidal Momentum27/1 -> Matrix Concatenate4/2
  Matrix Concatenate6/1 -> CMM/1
  Centroidal Momentum6/1 -> Matrix Concatenate3/1
  Centroidal Momentum8/1 -> Matrix Concatenate3/3
  Centroidal Momentum20/1 -> Matrix Concatenate1/5
  Centroidal Momentum11/1 -> Matrix Concatenate5/1
  jointPos/1 -> Centroidal Momentum22/2, Centroidal Momentum23/2, Centroidal Momentum24/2, Centroidal Momentum31/2, Centroidal Momentum25/2, Centroidal Momentum21/2, Centroidal Momentum16/2, Centroidal Momentum20/2, Centroidal Momentum19/2, Centroidal Momentum18/2, Centroidal Momentum17/2, Centroidal Momentum1/2, Centroidal Momentum2/2, Centroidal Momentum5/2, Centroidal Momentum4/2, Centroidal Momentum3/2, Centroidal Momentum10/2, Centroidal Momentum9/2, Centroidal Momentum8/2, Centroidal Momentum7/2, Centroidal Momentum6/2, Centroidal Momentum15/2, Centroidal Momentum14/2, Centroidal Momentum13/2, Centroidal Momentum11/2, Centroidal Momentum12/2, Centroidal Momentum30/2, Centroidal Momentum29/2, Centroidal Momentum28/2, Centroidal Momentum27/2, Centroidal Momentum26/2
  Matrix Concatenate2/1 -> Matrix Concatenate6/3
  Centroidal Momentum31/1 -> Matrix Concatenate/6
  Centroidal Momentum18/1 -> Matrix Concatenate1/3
  Constant36/1 -> Centroidal Momentum12/4
  Constant23/1 -> Centroidal Momentum11/4
  Constant6/1 -> Centroidal Momentum31/3
  Centroidal Momentum10/1 -> Matrix Concatenate3/5
  Constant18/1 -> Centroidal Momentum5/4
  Constant13/1 -> Centroidal Momentum20/4
  Constant/1 -> Centroidal Momentum21/3
  Constant28/1 -> Centroidal Momentum13/4
  Constant29/1 -> Centroidal Momentum14/4
  Constant1/1 -> Centroidal Momentum22/3
  Constant21/1 -> Centroidal Momentum9/4
  Centroidal Momentum16/1 -> Matrix Concatenate1/1
  Constant14/1 -> Centroidal Momentum1/4
  Constant10/1 -> Centroidal Momentum17/4
  Constant31/1 -> Centroidal Momentum26/4
  Constant8/1 -> Centroidal Momentum5/3, Centroidal Momentum4/3, Centroidal Momentum3/3, Centroidal Momentum2/3, Centroidal Momentum1/3
  Constant37/1 -> Centroidal Momentum23/3
  Constant5/1 -> Centroidal Momentum21/4, Centroidal Momentum22/4, Centroidal Momentum31/4, Centroidal Momentum25/4, Centroidal Momentum24/4, Centroidal Momentum23/4
  Constant22/1 -> Centroidal Momentum10/4
  Constant7/1 -> Centroidal Momentum20/3, Centroidal Momentum19/3, Centroidal Momentum18/3, Centroidal Momentum17/3, Centroidal Momentum16/3
  Constant16/1 -> Centroidal Momentum3/4
  Constant35/1 -> Centroidal Momentum30/4
  Constant12/1 -> Centroidal Momentum19/4
  Constant19/1 -> Centroidal Momentum6/4
  Constant11/1 -> Centroidal Momentum18/4
  Constant4/1 -> Centroidal Momentum25/3
  Constant9/1 -> Centroidal Momentum16/4
  Constant3/1 -> Centroidal Momentum24/3
  Constant32/1 -> Centroidal Momentum27/4
  Constant15/1 -> Centroidal Momentum2/4
  Centroidal Momentum13/1 -> Matrix Concatenate5/2
  Constant34/1 -> Centroidal Momentum29/4
  Constant24/1 -> Centroidal Momentum10/3, Centroidal Momentum9/3, Centroidal Momentum8/3, Centroidal Momentum7/3, Centroidal Momentum6/3
  Constant20/1 -> Centroidal Momentum7/4
  Constant25/1 -> Centroidal Momentum15/3, Centroidal Momentum14/3, Centroidal Momentum13/3, Centroidal Momentum11/3
  Centroidal Momentum9/1 -> Matrix Concatenate3/4
  Constant27/1 -> Centroidal Momentum8/4
  Centroidal Momentum17/1 -> Matrix Concatenate1/2
  Constant26/1 -> Centroidal Momentum12/3, Centroidal Momentum30/3, Centroidal Momentum29/3, Centroidal Momentum28/3, Centroidal Momentum27/3, Centroidal Momentum26/3
  Constant17/1 -> Centroidal Momentum4/4
  Constant30/1 -> Centroidal Momentum15/4
  Constant33/1 -> Centroidal Momentum28/4
  Centroidal Momentum30/1 -> Matrix Concatenate4/5
  Matrix Concatenate3/1 -> Matrix Concatenate6/4
  Centroidal Momentum22/1 -> Matrix Concatenate/2
  Centroidal Momentum21/1 -> Matrix Concatenate/1

== matlab function Flying Controller/stateDemuxFCN ==
  data: state input double; w_H_b output double; jointPos output double; baseTwist output double; jointVel output double; Config parameter double
function [w_H_b, jointPos, baseTwist, jointVel] = stateDemuxFCN(state, Config)

    [w_H_b, jointPos, baseTwist, jointVel] = stateDemux(state, Config);
end

== matlab function Flying Controller/comRefs/trajectoryGeneratorCoM ==
  settings: updateMethod=DISCRETE
  data: t input double; posCoM_0 input double; w_H_b_0 input double; posCoM_des output double; Config parameter double; rotationRef_base output double; velCoM_des output double; tSettling output double
function [posCoM_des, rotationRef_base, velCoM_des, tSettling] = referencesFCN(t, posCoM_0, w_H_b_0, Config)

    [posCoM_des, rotationRef_base, velCoM_des, tSettling] = references(t, posCoM_0, w_H_b_0, Config);
end

== matlab function Flying Controller/comRefs/Fake Holder2/MATLAB Function ==
  settings: updateMethod=DISCRETE
  data: s input double; s0 output double; unused input double
function s0 = fcn(s, ~)
persistent state
%#codegen

if isempty(state)
    state = s;
end

s0 = state;

== matlab function Flying Controller/matrixOfJetsAxes/axesOfJetsFCN ==
  data: w_H_J1 input double; matrixOfJetsAxes output double; w_H_J2 input double; w_H_J3 input double; w_H_J4 input double; posCoM input double; matrixOfJetsArms output double; Config parameter double
function [matrixOfJetsAxes, matrixOfJetsArms] = axesOfJetsFCN(w_H_J1, w_H_J2, w_H_J3, w_H_J4, posCoM, Config)

    [matrixOfJetsAxes, matrixOfJetsArms] = axesOfJets(w_H_J1, w_H_J2, w_H_J3, w_H_J4, posCoM, Config);
end

== matlab function Flying Controller/controller/controllerFlyingHumanoidsFCN ==
  data: jetsIntensities input double; matrixOfJetsAxes input double; matrixOfJetsArms input double; w_H_b input double; jointPos input double; jointPos_des input double; M_and_M_c input double; h_and_h_c input double; J_and_J_c input double; J_CoM input double; JDot_nu_and_JDot_nu_c input double; nu_and_nu_c input double; pos_vel_acc_CoM_des input double; L input double; intL input double; CMM_and_CMM_c input double; posCoM_des input double; rotationRef_base input double; hessianMatrixQP output double; gVectorQP output double; constraintMatA output double; lowerBoundQPMatA output double; upperBoundQPMatA output double; lowerBoundQP output double; upperBoundQP output double; Config parameter double; aux output double
function [hessianMatrixQP, gVectorQP, constraintMatA, lowerBoundQPMatA, upperBoundQPMatA, lowerBoundQP, upperBoundQP, aux] = ...
             controllerFCN(jetsIntensities, matrixOfJetsAxes, matrixOfJetsArms, w_H_b, jointPos, jointPos_des, M_and_M_c, h_and_h_c, J_and_J_c, J_CoM, JDot_nu_and_JDot_nu_c, nu_and_nu_c, pos_vel_acc_CoM_des, L, intL, CMM_and_CMM_c, posCoM_des, rotationRef_base, Config)

    [hessianMatrixQP, gVectorQP, constraintMatA, lowerBoundQPMatA, upperBoundQPMatA, lowerBoundQP, upperBoundQP, aux] = ...
        controller(jetsIntensities, matrixOfJetsAxes, matrixOfJetsArms, w_H_b, jointPos, jointPos_des, M_and_M_c, h_and_h_c, J_and_J_c, J_CoM, JDot_nu_and_JDot_nu_c, nu_and_nu_c, pos_vel_acc_CoM_des, L, intL, CMM_and_CMM_c, posCoM_des, rotationRef_base, Config);
end

== matlab function Robot Dynamics/fromStateToForces/matrixOfJetsAxes/axesOfJetsFCN ==
  data: w_H_J1 input double; matrixOfJetsAxes output double; w_H_J2 input double; w_H_J3 input double; w_H_J4 input double; posCoM input double; matrixOfJetsArms output double; Config parameter double
function [matrixOfJetsAxes, matrixOfJetsArms] = axesOfJetsFCN(w_H_J1, w_H_J2, w_H_J3, w_H_J4, posCoM, Config)

    [matrixOfJetsAxes, matrixOfJetsArms] = axesOfJets(w_H_J1, w_H_J2, w_H_J3, w_H_J4, posCoM, Config);
end

== matlab function Flying Controller/controller/torqueControl ==
  data: jetsIntensities input double; matrixOfJetsAxes input double; jointVel_des input double; M_and_M_c input double; J_and_J_c input double; h_and_h_c input double; nu_and_nu_c input double; intTildeDot input double; jointTorques output double; Config parameter double; jointVel_err output double
function [jointTorques, jointVel_err] = torqueControlFCN(jetsIntensities, matrixOfJetsAxes, jointVel_des, M_and_M_c, J_and_J_c, h_and_h_c, nu_and_nu_c, intTildeDot, Config)

    [jointTorques, jointVel_err] = torqueControl(jetsIntensities, matrixOfJetsAxes, jointVel_des, M_and_M_c, h_and_h_c, J_and_J_c, nu_and_nu_c, intTildeDot, Config);
end

== matlab function Visualizer/transpose1 ==
  data: momentum input double; w_H_b input double; rotBaseDes input double; orientationError output double; angularMomentum output double
function [orientationError, angularMomentum] = norm(momentum, w_H_b, rotBaseDes)

    orientationError = norm(rotBaseDes(1:3,1:3)'*w_H_b(1:3,1:3)-eye(3));
    angularMomentum  = norm(momentum(4:6));
end

== matlab function Robot Dynamics/Robot Dynamics ==
  settings: updateMethod=DISCRETE
  data: M input double; h input double; J input double; f input double; tau input double; state input double; stateDot output double; Config parameter double
function stateDot = robotDynamicsFCN(M, h, J, f, tau, state, Config)

    stateDot = dynamics(M, h, J, f, tau, state, Config);
end

== matlab function Robot Dynamics/fromStateToForces/fromJetsIntensitiesToForces ==
  data: matrixOfJetsAxes input double; jetsIntensities input double; f output double
function f = fromJetsIntensitiesToForcesFCN(matrixOfJetsAxes, jetsIntensities)

    f = fromJetsIntensitiesToForces(matrixOfJetsAxes, jetsIntensities);
end

== matlab function Robot Dynamics/stateDemuxFCN ==
  settings: updateMethod=DISCRETE
  data: state input double; w_H_b output double; jointPos output double; baseTwist output double; jointVel output double; Config parameter double
function [w_H_b, jointPos, baseTwist, jointVel] = stateDemuxFCN(state, Config)

    [w_H_b, jointPos, baseTwist, jointVel] = stateDemux(state, Config);
end

== matlab function Flying Controller/controller/Evaluate initial jets intensities ==
  data: matrixOfJetsAxes input double; M_and_M_c input double; J_and_J_c input double; pos_vel_acc_CoM_des input double; j_0 output double; Config parameter double
function   j_0 = jetIntensitiesAtZeroFCN(matrixOfJetsAxes, M_and_M_c, J_and_J_c, pos_vel_acc_CoM_des, Config)

    j_0 = jetIntensitiesAtZero(matrixOfJetsAxes, M_and_M_c, J_and_J_c, pos_vel_acc_CoM_des, Config);
end

== matlab function Flying Controller/controller/transpose1 ==
  data: u input double; norm_u output double
function norm_u = norm(u)

   norm_u = norm(u);
end

== matlab function Flying Controller/comRefs/Fake Holder1/MATLAB Function ==
  settings: updateMethod=DISCRETE
  data: s input double; s0 output double; unused input double
function s0 = fcn(s, ~)
persistent state
%#codegen

if isempty(state)
    state = s;
end

s0 = state;

== matlab function Flying Controller/Dynamics and Kinematics/fromFloatingToCentroidalDynamics/fromFloating2Centroidal ==
  data: M input double; M_c output double; h input double; g input double; J input double; JDot_nu input double; nu input double; c_T_b input double; TDot input double; h_c output double; J_c output double; JDot_nu_c output double; nu_c output double; CMM output double; CMM_c output double
function [M_c, h_c, J_c, JDot_nu_c, nu_c, CMM, CMM_c] = fromFloatingToCentroidalDynamicsFCN(M, h, g, J, JDot_nu, nu, c_T_b, TDot)

    [M_c, h_c, J_c, JDot_nu_c, nu_c, CMM, CMM_c] = fromFloatingToCentroidalDynamics(M, h, g, J, JDot_nu, nu, c_T_b, TDot);
end
